simulink model "BLDCMODELTOTALNEURON"  (R2020a)
settings: Solver=ode45  StartTime=0.0  StopTime=2  RelTol=1e-3  EnableMultiTasking=on
InitFcn:
  | clc;
StopFcn:
  | clc;
undefined symbols (not defined in the file): sigbuilder_block, Ts
libraries: neural x55, fl_lib x14, nesl_utility x14, simulink x7, spsIGBTDiodeLib x6, spsVoltageMeasurementLib x3, powerlib_extras x1, spsControlledVoltageSourceLib x1, spsGroundLib x1, spsThreePhaseVIMeasurementLib x1, spspowerguiLib x1
(part 2 of 3)

== system BLDCMODELTOTALNEURON/BLDC Model/emf generation/Phase c ==
  note: Phi' r
  the,we : Inport
  Demux : Demux  Outputs=2
      settings: DisplayOption=none
  Gain4 : Gain  Gain=0.175  SaturateOnIntegerOverflow=on  OutDataTypeStr=Inherit: Same as input  ParamDataTypeStr=Inherit: Same as input
  Product1 : Product  SaturateOnIntegerOverflow=on  OutDataTypeStr=Inherit: Same as first input
  cos (u(1)) : Subsystem
  phi'r : Outport
  E : Outport  Port=2
  wires:
  Gain4/1 -> Product1/1, phi'r/1
  Product1/1 -> E/1
  the,we/1 -> Demux/1
  Demux/2 -> Product1/2
  Demux/1 -> cos (u(1))/1(In1)
  cos (u(1))/1(Out1) -> Gain4/1

== system BLDCMODELTOTALNEURON/Function Fitting Neural Network/Layer 1/Delays 1 ==
  "p{1}" : Inport  PortDimensions=9
      mask Display: e = 0.06;c1 = [120 230 180]/255;c2 = ([120 230 180]+0)/(256+128);c3 = ([120 230 180]+128)/(256+128);patch([0 1 1 0],[0 0 1 1],c1);patch([0 1 1 1-e 1-e 0+e],[0 0 1 1-e 0+e 0+e],c2);patch([0 0 1 1-e 0+e 0+e],[0 1 1 1-e 1-e 0+e],c3);plot([0 1 1 0 0],[0 0 1 1 0]);
  mux : Mux  Inputs=1
      mask Display: e = 0.06;c1 = [120 150 230]/255;c2 = ([120 150 230]+0)/383;c3 = ([120 150 230]+128)/383;patch([0 1 1 0],[0 0 1 1],c1);patch([0 1 1 1-e 1-e 0+e],[0 0 1 1-e 0+e 0+e],c2);patch([0 0 1 1-e 0+e 0+e],[0 1 1 1-e 1-e 0+e],c3);plot([0 1 1 0 0],[0 0 1 1 0]);disp('Mux')
  "pd{1,1}" : Outport
      mask Display: e = 0.06;c1 = [120 230 180]/255;c2 = ([120 230 180]+0)/(256+128);c3 = ([120 230 180]+128)/(256+128);patch([0 1 1 0],[0 0 1 1],c1);patch([0 1 1 1-e 1-e 0+e],[0 0 1 1-e 0+e 0+e],c2);patch([0 0 1 1-e 0+e 0+e],[0 1 1 1-e 1-e 0+e],c3);plot([0 1 1 0 0],[0 0 1 1 0]);
  wires:
  "p{1}"/1 -> mux/1
  mux/1 -> "pd{1,1}"/1

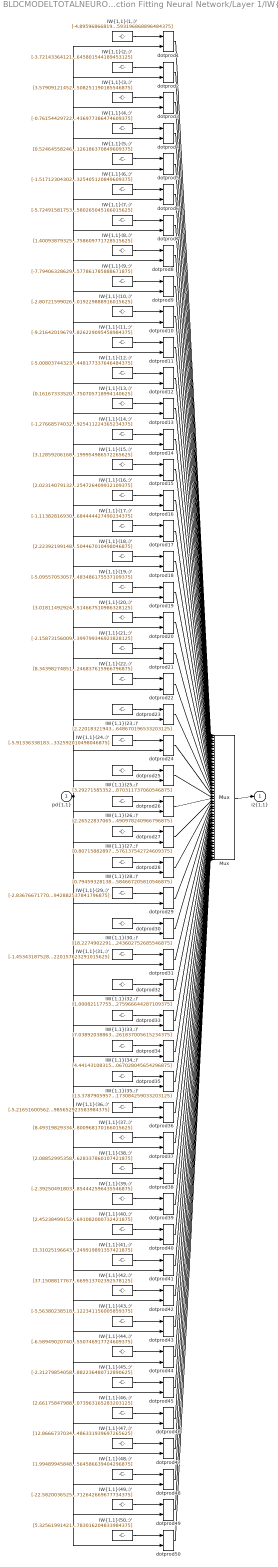
== system BLDCMODELTOTALNEURON/Function Fitting Neural Network/Layer 1/IW{1,1} ==
  "pd{1,1}" : Inport  PortDimensions=9
      mask Display: e = 0.06;c1 = [120 230 180]/255;c2 = ([120 230 180]+0)/(256+128);c3 = ([120 230 180]+128)/(256+128);patch([0 1 1 0],[0 0 1 1],c1);patch([0 1 1 1-e 1-e 0+e],[0 0 1 1-e 0+e 0+e],c2);patch([0 0 1 1-e 0+e 0+e],[0 1 1 1-e 1-e 0+e],c3);plot([0 1 1 0 0],[0 0 1 1 0]);
  "IW{1,1}(1,:)'" : Constant  Value=[-4.895968668193777517672060639597475528717041015625;5.40347313688422303812330937944352626800537109375;2.74044730962565186160873054177500307559967041015625;2.61285690437117157358670738176442682743072509765625;-8.18219538608644114674461889080703258514404296875;5.37405300526213380862827762030065059661865234375;-2.547081241809125540243030627607367932796478271484375;-7.45222912554785299477089210995472967624664306640625;2.3353386247630023575538871227763593196868896484375]
      mask Display: e = 0.06;c1 = [120 150 230]/255;c2 = ([120 150 230]+0)/383;c3 = ([120 150 230]+128)/383;patch([0 1 1 0],[0 0 1 1],c1);patch([0 1 1 1-e 1-e 0+e],[0 0 1 1-e 0+e 0+e],c2);patch([0 0 1 1-e 0+e 0+e],[0 1 1 1-e 1-e 0+e],c3);plot([0 1 1 0 0],[0 0 1 1 0]);disp('Weights');
  "IW{1,1}(10,:)'" : Constant  Value=[-2.807215990265720773066959736752323806285858154296875;0.53318125450332398695962865531328134238719940185546875;1.73233750776441564056540300953201949596405029296875;-6.7636512082147479674176793196238577365875244140625;6.88789031656800165848153483239002525806427001953125;-1.1843020529516923300406006092089228332042694091796875;1.77424013763668231291603660793043673038482666015625;7.99713610623197279636542589287273585796356201171875;0.447326594167716307115512108794064261019229888916015625]
      mask Display: e = 0.06;c1 = [120 150 230]/255;c2 = ([120 150 230]+0)/383;c3 = ([120 150 230]+128)/383;patch([0 1 1 0],[0 0 1 1],c1);patch([0 1 1 1-e 1-e 0+e],[0 0 1 1-e 0+e 0+e],c2);patch([0 0 1 1-e 0+e 0+e],[0 1 1 1-e 1-e 0+e],c3);plot([0 1 1 0 0],[0 0 1 1 0]);disp('Weights');
  "IW{1,1}(11,:)'" : Constant  Value=[-9.216420196795439778725267387926578521728515625;7.1594195626589272052342494134791195392608642578125;3.118246074238363529929074502433650195598602294921875;0.74384522324622814881678323217784054577350616455078125;-2.420490963926231753333695451146923005580902099609375;5.44455711163404476593541403417475521564483642578125;3.547825214125399639897295855917036533355712890625;4.30621318872842895331132240244187414646148681640625;1.096405026223636891558044226258061826229095458984375]
      mask Display: e = 0.06;c1 = [120 150 230]/255;c2 = ([120 150 230]+0)/383;c3 = ([120 150 230]+128)/383;patch([0 1 1 0],[0 0 1 1],c1);patch([0 1 1 1-e 1-e 0+e],[0 0 1 1-e 0+e 0+e],c2);patch([0 0 1 1-e 0+e 0+e],[0 1 1 1-e 1-e 0+e],c3);plot([0 1 1 0 0],[0 0 1 1 0]);disp('Weights');
  "IW{1,1}(12,:)'" : Constant  Value=[-5.00803744323493038592687298660166561603546142578125;5.9761920590233188477213843725621700286865234375;0.320001378281075166132296772047993727028369903564453125;-2.738915566294051640028328620246611535549163818359375;1.0574131975688112472511193118407391011714935302734375;11.1576349013176656654877660912461578845977783203125;10.25816732987643575825131847523152828216552734375;5.71739885726999741422105216770432889461517333984375;0.52981483115273331208072704612277448177337646484375]
      mask Display: e = 0.06;c1 = [120 150 230]/255;c2 = ([120 150 230]+0)/383;c3 = ([120 150 230]+128)/383;patch([0 1 1 0],[0 0 1 1],c1);patch([0 1 1 1-e 1-e 0+e],[0 0 1 1-e 0+e 0+e],c2);patch([0 0 1 1-e 0+e 0+e],[0 1 1 1-e 1-e 0+e],c3);plot([0 1 1 0 0],[0 0 1 1 0]);disp('Weights');
  "IW{1,1}(13,:)'" : Constant  Value=[0.1616733352080349794821501063779578544199466705322265625;-1.90626528235715131387451037880964577198028564453125;1.1517495220095372854274273777264170348644256591796875;-1.468598245944300106913260606233961880207061767578125;-6.27844796813521188738604905665852129459381103515625;3.5109383197600099180135657661594450473785400390625;-3.687189907329767368793227433343417942523956298828125;-1.6200010345593092164762083484674803912639617919921875;2.260455325759112898964531268575228750705718994140625]
      mask Display: e = 0.06;c1 = [120 150 230]/255;c2 = ([120 150 230]+0)/383;c3 = ([120 150 230]+128)/383;patch([0 1 1 0],[0 0 1 1],c1);patch([0 1 1 1-e 1-e 0+e],[0 0 1 1-e 0+e 0+e],c2);patch([0 0 1 1-e 0+e 0+e],[0 1 1 1-e 1-e 0+e],c3);plot([0 1 1 0 0],[0 0 1 1 0]);disp('Weights');
  "IW{1,1}(14,:)'" : Constant  Value=[-1.2766857403284517236130568562657572329044342041015625;-5.73369882955798715329365222714841365814208984375;3.227374843555661954042079742066562175750732421875;-7.7809955575162117469290024018846452236175537109375;2.80775474671538471937992653693072497844696044921875;-4.3767986431355172527446484309621155261993408203125;7.8290605045435910369633347727358341217041015625;6.4679041165319812733969229157082736492156982421875;-3.894484835375331410745047833188436925411224365234375]
      mask Display: e = 0.06;c1 = [120 150 230]/255;c2 = ([120 150 230]+0)/383;c3 = ([120 150 230]+128)/383;patch([0 1 1 0],[0 0 1 1],c1);patch([0 1 1 1-e 1-e 0+e],[0 0 1 1-e 0+e 0+e],c2);patch([0 0 1 1-e 0+e 0+e],[0 1 1 1-e 1-e 0+e],c3);plot([0 1 1 0 0],[0 0 1 1 0]);disp('Weights');
  "IW{1,1}(15,:)'" : Constant  Value=[3.1285920616828253315588881378062069416046142578125;2.81705887052771064560374725260771811008453369140625;-3.887956696466934314315722076571546494960784912109375;5.02906629611409972113733601872809231281280517578125;0.6170228014013081629940415950841270387172698974609375;4.6865213003801642344114952720701694488525390625;-8.101108360563227250850104610435664653778076171875;-4.9140036575473029500926713808439671993255615234375;4.058733138775412641052753315307199954986572265625]
      mask Display: e = 0.06;c1 = [120 150 230]/255;c2 = ([120 150 230]+0)/383;c3 = ([120 150 230]+128)/383;patch([0 1 1 0],[0 0 1 1],c1);patch([0 1 1 1-e 1-e 0+e],[0 0 1 1-e 0+e 0+e],c2);patch([0 0 1 1-e 0+e 0+e],[0 1 1 1-e 1-e 0+e],c3);plot([0 1 1 0 0],[0 0 1 1 0]);disp('Weights');
  "IW{1,1}(16,:)'" : Constant  Value=[2.023140791325761522756465637939982116222381591796875;3.199313205814582783403920984710566699504852294921875;-3.629430220216549596301547353505156934261322021484375;2.30078335496623598288579159998334944248199462890625;-3.870890427542229783597349523915909230709075927734375;2.513060115012128559186521670198999345302581787109375;-2.583375254625132289021394171868450939655303955078125;-4.177607392620398485405530664138495922088623046875;-0.476403165367220216008803390650427900254726409912109375]
      mask Display: e = 0.06;c1 = [120 150 230]/255;c2 = ([120 150 230]+0)/383;c3 = ([120 150 230]+128)/383;patch([0 1 1 0],[0 0 1 1],c1);patch([0 1 1 1-e 1-e 0+e],[0 0 1 1-e 0+e 0+e],c2);patch([0 0 1 1-e 0+e 0+e],[0 1 1 1-e 1-e 0+e],c3);plot([0 1 1 0 0],[0 0 1 1 0]);disp('Weights');
  "IW{1,1}(17,:)'" : Constant  Value=[-1.113828169301168458105166791938245296478271484375;1.1778404473012773490125937314587645232677459716796875;1.620901404126910971825736851315014064311981201171875;-1.766146228500121484472629163064993917942047119140625;0.646115936343579999601161034661345183849334716796875;1.66630542385350910450370065518654882907867431640625;1.2524116425207412195419465206214226782321929931640625;0.8812841366291574995983637563767842948436737060546875;2.343840383667620042018597814603708684444427490234375]
      mask Display: e = 0.06;c1 = [120 150 230]/255;c2 = ([120 150 230]+0)/383;c3 = ([120 150 230]+128)/383;patch([0 1 1 0],[0 0 1 1],c1);patch([0 1 1 1-e 1-e 0+e],[0 0 1 1-e 0+e 0+e],c2);patch([0 0 1 1-e 0+e 0+e],[0 1 1 1-e 1-e 0+e],c3);plot([0 1 1 0 0],[0 0 1 1 0]);disp('Weights');
  "IW{1,1}(18,:)'" : Constant  Value=[2.223921991486593530140680741169489920139312744140625;-0.054825426871896072722467607718499493785202503204345703125;0.0022185476097710652050587487593702462618239223957061767578125;-0.5843966860481921710146480108960531651973724365234375;3.799990339256197557915584184229373931884765625;-1.9218355438914278554562997669563628733158111572265625;-3.537447672391386799262136264587752521038055419921875;-1.0586896092735147423269381761201657354831695556640625;2.684374086787240099027940232190303504467010498046875]
      mask Display: e = 0.06;c1 = [120 150 230]/255;c2 = ([120 150 230]+0)/383;c3 = ([120 150 230]+128)/383;patch([0 1 1 0],[0 0 1 1],c1);patch([0 1 1 1-e 1-e 0+e],[0 0 1 1-e 0+e 0+e],c2);patch([0 0 1 1-e 0+e 0+e],[0 1 1 1-e 1-e 0+e],c3);plot([0 1 1 0 0],[0 0 1 1 0]);disp('Weights');
  "IW{1,1}(19,:)'" : Constant  Value=[-5.0955705305759071421789485611952841281890869140625;6.05178194090348053890693336143158376216888427734375;-1.491669072534929085804833448491990566253662109375;-0.94100410130936185115757552921422757208347320556640625;-1.6970243036780334744406673053163103759288787841796875;-2.266366636401446754689459339715540409088134765625;-3.1732804450517395622455296688713133335113525390625;2.774317765718105288641481820377521216869354248046875;1.1986759118675640589657405143952928483486175537109375]
      mask Display: e = 0.06;c1 = [120 150 230]/255;c2 = ([120 150 230]+0)/383;c3 = ([120 150 230]+128)/383;patch([0 1 1 0],[0 0 1 1],c1);patch([0 1 1 1-e 1-e 0+e],[0 0 1 1-e 0+e 0+e],c2);patch([0 0 1 1-e 0+e 0+e],[0 1 1 1-e 1-e 0+e],c3);plot([0 1 1 0 0],[0 0 1 1 0]);disp('Weights');
  "IW{1,1}(2,:)'" : Constant  Value=[-3.7214336412183417479582203668542206287384033203125;8.4268142416087190582629773416556417942047119140625;-3.02879148438673073684412884176708757877349853515625;0.2284576077078076250526095236637047491967678070068359375;1.005184022489817419199198411661200225353240966796875;4.73916034710702316345987128443084657192230224609375;2.513388967630310499856705064303241670131683349609375;-2.5965278619095233381131038186140358448028564453125;-4.3974879944557887512246452388353645801544189453125]
      mask Display: e = 0.06;c1 = [120 150 230]/255;c2 = ([120 150 230]+0)/383;c3 = ([120 150 230]+128)/383;patch([0 1 1 0],[0 0 1 1],c1);patch([0 1 1 1-e 1-e 0+e],[0 0 1 1-e 0+e 0+e],c2);patch([0 0 1 1-e 0+e 0+e],[0 1 1 1-e 1-e 0+e],c3);plot([0 1 1 0 0],[0 0 1 1 0]);disp('Weights');
  "IW{1,1}(20,:)'" : Constant  Value=[3.01811492924852498020982238813303411006927490234375;-3.62725956127743831558518650126643478870391845703125;-1.842623857170338386168850774993188679218292236328125;-5.19975075112496920581861559185199439525604248046875;1.966417547133222143429520656354725360870361328125;0.2434354388569480998061322907233261503279209136962890625;8.19305073136916917064809240400791168212890625;0.87614260508461594412210615701042115688323974609375;-0.89756050648464213992383520235307514667510986328125]
      mask Display: e = 0.06;c1 = [120 150 230]/255;c2 = ([120 150 230]+0)/383;c3 = ([120 150 230]+128)/383;patch([0 1 1 0],[0 0 1 1],c1);patch([0 1 1 1-e 1-e 0+e],[0 0 1 1-e 0+e 0+e],c2);patch([0 0 1 1-e 0+e 0+e],[0 1 1 1-e 1-e 0+e],c3);plot([0 1 1 0 0],[0 0 1 1 0]);disp('Weights');
  "IW{1,1}(21,:)'" : Constant  Value=[-2.158731560096526447267706316779367625713348388671875;-0.8746332604844859748283170119975693523883819580078125;3.05676503556049272702921371092088520526885986328125;3.081958001652896239619394691544584929943084716796875;-6.09089804270805057484494682285003364086151123046875;-1.5170091317769973660034565909882076084613800048828125;2.515311414585273297461753827519714832305908203125;-1.51894932821134087674863621941767632961273193359375;4.67491695196711010140688813407905399799346923828125]
      mask Display: e = 0.06;c1 = [120 150 230]/255;c2 = ([120 150 230]+0)/383;c3 = ([120 150 230]+128)/383;patch([0 1 1 0],[0 0 1 1],c1);patch([0 1 1 1-e 1-e 0+e],[0 0 1 1-e 0+e 0+e],c2);patch([0 0 1 1-e 0+e 0+e],[0 1 1 1-e 1-e 0+e],c3);plot([0 1 1 0 0],[0 0 1 1 0]);disp('Weights');
  "IW{1,1}(22,:)'" : Constant  Value=[8.343982748517642988872466958127915859222412109375;-2.161196645266016513886597749660722911357879638671875;-3.9544004180846030749307828955352306365966796875;-2.43457845164129249582174452370963990688323974609375;-5.205305155843110043178967316634953022003173828125;1.0130992099416860074967416949220933020114898681640625;6.34578855801143770776207020389847457408905029296875;2.20944537619115966009530893643386662006378173828125;-0.484853150291399248583701364623266272246837615966796875]
      mask Display: e = 0.06;c1 = [120 150 230]/255;c2 = ([120 150 230]+0)/383;c3 = ([120 150 230]+128)/383;patch([0 1 1 0],[0 0 1 1],c1);patch([0 1 1 1-e 1-e 0+e],[0 0 1 1-e 0+e 0+e],c2);patch([0 0 1 1-e 0+e 0+e],[0 1 1 1-e 1-e 0+e],c3);plot([0 1 1 0 0],[0 0 1 1 0]);disp('Weights');
  "IW{1,1}(23,:)'" : Constant  Value=[2.22018321943891461245357277221046388149261474609375;-1.8800292969605318926795689549180679023265838623046875;-2.243768721796227882947505349875427782535552978515625;-1.057276982754526084562485266360454261302947998046875;-1.2433812829791133225398880313150584697723388671875;-1.383969860461479850499699750798754394054412841796875;3.058730398982790976702972329803742468357086181640625;0.53913955545679181913243382950895465910434722900390625;0.1595438162536411408343184348268550820648670196533203125]
      mask Display: e = 0.06;c1 = [120 150 230]/255;c2 = ([120 150 230]+0)/383;c3 = ([120 150 230]+128)/383;patch([0 1 1 0],[0 0 1 1],c1);patch([0 1 1 1-e 1-e 0+e],[0 0 1 1-e 0+e 0+e],c2);patch([0 0 1 1-e 0+e 0+e],[0 1 1 1-e 1-e 0+e],c3);plot([0 1 1 0 0],[0 0 1 1 0]);disp('Weights');
  "IW{1,1}(24,:)'" : Constant  Value=[-5.9133633818331219345054705627262592315673828125;7.325130508331572087854510755278170108795166015625;0.67854478523987860061339461026364006102085113525390625;-5.54971457443748494853252850589342415332794189453125;2.338297073162864503359514856128953397274017333984375;-4.82297855274858289220674123498611152172088623046875;4.53075163897600052820280325249768793582916259765625;7.4605392659156422041633049957454204559326171875;-0.129756839337727025718294271428021602332592010498046875]
      mask Display: e = 0.06;c1 = [120 150 230]/255;c2 = ([120 150 230]+0)/383;c3 = ([120 150 230]+128)/383;patch([0 1 1 0],[0 0 1 1],c1);patch([0 1 1 1-e 1-e 0+e],[0 0 1 1-e 0+e 0+e],c2);patch([0 0 1 1-e 0+e 0+e],[0 1 1 1-e 1-e 0+e],c3);plot([0 1 1 0 0],[0 0 1 1 0]);disp('Weights');
  "IW{1,1}(25,:)'" : Constant  Value=[3.2927158535273175488100605434738099575042724609375;-7.466663455404482618860129150561988353729248046875;1.859971234331494915892335484386421740055084228515625;-4.40535563617537917480149189941585063934326171875;-1.4389465848187310559325169379008002579212188720703125;-7.14086549853874519300234169350005686283111572265625;13.11373443627413593048913753591477870941162109375;2.926398481880311042147013722569681704044342041015625;-4.11809256079247898441053621354512870311737060546875]
      mask Display: e = 0.06;c1 = [120 150 230]/255;c2 = ([120 150 230]+0)/383;c3 = ([120 150 230]+128)/383;patch([0 1 1 0],[0 0 1 1],c1);patch([0 1 1 1-e 1-e 0+e],[0 0 1 1-e 0+e 0+e],c2);patch([0 0 1 1-e 0+e 0+e],[0 1 1 1-e 1-e 0+e],c3);plot([0 1 1 0 0],[0 0 1 1 0]);disp('Weights');
  "IW{1,1}(26,:)'" : Constant  Value=[2.26522837065874060868964079418219625949859619140625;4.2525822507105086600631693727336823940277099609375;-4.61264142259110609955996551434509456157684326171875;-6.31738226144889036817176020122133195400238037109375;5.23253833887288255510839007911272346973419189453125;-8.962684825422229550895281136035919189453125;-5.88140626410156119874272917513735592365264892578125;6.1683261761612886431294100475497543811798095703125;-5.83295418242180829793142038397490978240966796875]
      mask Display: e = 0.06;c1 = [120 150 230]/255;c2 = ([120 150 230]+0)/383;c3 = ([120 150 230]+128)/383;patch([0 1 1 0],[0 0 1 1],c1);patch([0 1 1 1-e 1-e 0+e],[0 0 1 1-e 0+e 0+e],c2);patch([0 0 1 1-e 0+e 0+e],[0 1 1 1-e 1-e 0+e],c3);plot([0 1 1 0 0],[0 0 1 1 0]);disp('Weights');
  "IW{1,1}(27,:)'" : Constant  Value=[0.80715882897217128277844722106237895786762237548828125;-1.5342936386238827939365592101239599287509918212890625;-0.42012466949483495692874157612095586955547332763671875;-8.11645473537303274724763468839228153228759765625;-1.1314757465724880614033054371247999370098114013671875;14.781667595466473130727536045014858245849609375;1.8109771676627250958091508437064476311206817626953125;3.9085959869213322548375799669884145259857177734375;-6.07921746579665178700224714702926576137542724609375]
      mask Display: e = 0.06;c1 = [120 150 230]/255;c2 = ([120 150 230]+0)/383;c3 = ([120 150 230]+128)/383;patch([0 1 1 0],[0 0 1 1],c1);patch([0 1 1 1-e 1-e 0+e],[0 0 1 1-e 0+e 0+e],c2);patch([0 0 1 1-e 0+e 0+e],[0 1 1 1-e 1-e 0+e],c3);plot([0 1 1 0 0],[0 0 1 1 0]);disp('Weights');
  "IW{1,1}(28,:)'" : Constant  Value=[0.79459328138242157901771633987664245069026947021484375;-1.8079929837847250606586158028221689164638519287109375;1.69049420812355766230439257924444973468780517578125;-0.73313934220313348166797595695243217051029205322265625;-1.5224778868556130273503868011175654828548431396484375;0.4887267103351027319746435750857926905155181884765625;3.311316422988955121553544813650660216808319091796875;0.575415043139363202584490863955579698085784912109375;-3.7366302997256735096698321285657584667205810546875]
      mask Display: e = 0.06;c1 = [120 150 230]/255;c2 = ([120 150 230]+0)/383;c3 = ([120 150 230]+128)/383;patch([0 1 1 0],[0 0 1 1],c1);patch([0 1 1 1-e 1-e 0+e],[0 0 1 1-e 0+e 0+e],c2);patch([0 0 1 1-e 0+e 0+e],[0 1 1 1-e 1-e 0+e],c3);plot([0 1 1 0 0],[0 0 1 1 0]);disp('Weights');
  "IW{1,1}(29,:)'" : Constant  Value=[-2.83676671770210919731880494509823620319366455078125;3.78002105566060198071909326245076954364776611328125;-2.323486567515789857907293480820953845977783203125;-0.95512967653330071993167393884505145251750946044921875;-0.60568244848216823417175191934802569448947906494140625;2.210703505491417697470524217351339757442474365234375;-2.039411367259091445447438672999851405620574951171875;-0.73412589888445289876273136542295105755329132080078125;-1.7846661191017278991211014727014116942882537841796875]
      mask Display: e = 0.06;c1 = [120 150 230]/255;c2 = ([120 150 230]+0)/383;c3 = ([120 150 230]+128)/383;patch([0 1 1 0],[0 0 1 1],c1);patch([0 1 1 1-e 1-e 0+e],[0 0 1 1-e 0+e 0+e],c2);patch([0 0 1 1-e 0+e 0+e],[0 1 1 1-e 1-e 0+e],c3);plot([0 1 1 0 0],[0 0 1 1 0]);disp('Weights');
  "IW{1,1}(3,:)'" : Constant  Value=[3.579091214525738084972772412584163248538970947265625;-2.431777730337249199266125287977047264575958251953125;-1.4837016201098738310548696972546167671680450439453125;3.025023954173181817139948179828934371471405029296875;-5.09547170650127778657179078436456620693206787109375;-4.7348999293881117722548879100941121578216552734375;-0.428598247009314980981997678100015036761760711669921875;-3.530088208951525086121137064765207469463348388671875;8.6702058743657044459496319177560508251190185546875]
      mask Display: e = 0.06;c1 = [120 150 230]/255;c2 = ([120 150 230]+0)/383;c3 = ([120 150 230]+128)/383;patch([0 1 1 0],[0 0 1 1],c1);patch([0 1 1 1-e 1-e 0+e],[0 0 1 1-e 0+e 0+e],c2);patch([0 0 1 1-e 0+e 0+e],[0 1 1 1-e 1-e 0+e],c3);plot([0 1 1 0 0],[0 0 1 1 0]);disp('Weights');
  "IW{1,1}(30,:)'" : Constant  Value=[18.2274902291847951119052595458924770355224609375;0.10029042444976567216574636631776229478418827056884765625;-15.2216980933245960017075049108825623989105224609375;-51.1700178399161842435205471701920032501220703125;-56.02455973781388109955514664761722087860107421875;47.243740956707284794902079738676548004150390625;10.6716383101642922071050634258426725864410400390625;27.839487972618687905423939810134470462799072265625;-6.3769331352299314374931782367639243602752685546875]
      mask Display: e = 0.06;c1 = [120 150 230]/255;c2 = ([120 150 230]+0)/383;c3 = ([120 150 230]+128)/383;patch([0 1 1 0],[0 0 1 1],c1);patch([0 1 1 1-e 1-e 0+e],[0 0 1 1-e 0+e 0+e],c2);patch([0 0 1 1-e 0+e 0+e],[0 1 1 1-e 1-e 0+e],c3);plot([0 1 1 0 0],[0 0 1 1 0]);disp('Weights');
  "IW{1,1}(31,:)'" : Constant  Value=[-1.4534318752841068889125608620815910398960113525390625;6.1247562160562427635568383266218006610870361328125;-2.8918337539965239813000152935273945331573486328125;0.9028102978327281480375177125097252428531646728515625;-4.3042053734154190891558755538426339626312255859375;-1.845935973018257403310826703091152012348175048828125;2.573811245121011115344344943878240883350372314453125;-3.919961580962290526031210902146995067596435546875;2.665708563941960651533236159593798220157623291015625]
      mask Display: e = 0.06;c1 = [120 150 230]/255;c2 = ([120 150 230]+0)/383;c3 = ([120 150 230]+128)/383;patch([0 1 1 0],[0 0 1 1],c1);patch([0 1 1 1-e 1-e 0+e],[0 0 1 1-e 0+e 0+e],c2);patch([0 0 1 1-e 0+e 0+e],[0 1 1 1-e 1-e 0+e],c3);plot([0 1 1 0 0],[0 0 1 1 0]);disp('Weights');
  "IW{1,1}(32,:)'" : Constant  Value=[1.000821177556808994069115215097554028034210205078125;-1.1601853380740809740245822467841207981109619140625;-1.2470947311945967950208569163805805146694183349609375;-1.288548983066672537489694150281138718128204345703125;1.099069146087539028400215102010406553745269775390625;-2.518438507999196218634097022004425525665283203125;7.2023214000541369017582837841473519802093505859375;5.20235982672458963094186401576735079288482666015625;-1.8693746816614795758226819089031778275966644287109375]
      mask Display: e = 0.06;c1 = [120 150 230]/255;c2 = ([120 150 230]+0)/383;c3 = ([120 150 230]+128)/383;patch([0 1 1 0],[0 0 1 1],c1);patch([0 1 1 1-e 1-e 0+e],[0 0 1 1-e 0+e 0+e],c2);patch([0 0 1 1-e 0+e 0+e],[0 1 1 1-e 1-e 0+e],c3);plot([0 1 1 0 0],[0 0 1 1 0]);disp('Weights');
  "IW{1,1}(33,:)'" : Constant  Value=[7.03892038863087776690008467994630336761474609375;-11.064903976837282328915534890256822109222412109375;0.69971359527199628036697731658932752907276153564453125;-6.25767087593949344892507724580354988574981689453125;1.2295683633822871438923129971954040229320526123046875;-22.917965838783505461151435156352818012237548828125;-0.1913542269049568200767197367895278148353099822998046875;-17.30670372769272802315754233859479427337646484375;-9.9208972492461295900056938990019261837005615234375]
      mask Display: e = 0.06;c1 = [120 150 230]/255;c2 = ([120 150 230]+0)/383;c3 = ([120 150 230]+128)/383;patch([0 1 1 0],[0 0 1 1],c1);patch([0 1 1 1-e 1-e 0+e],[0 0 1 1-e 0+e 0+e],c2);patch([0 0 1 1-e 0+e 0+e],[0 1 1 1-e 1-e 0+e],c3);plot([0 1 1 0 0],[0 0 1 1 0]);disp('Weights');
  "IW{1,1}(34,:)'" : Constant  Value=[4.44143108315375911843148060142993927001953125;1.5265309562414410837760669892304576933383941650390625;-4.78652973989852625891217030584812164306640625;2.7260670293901849703388506895862519741058349609375;-0.1258984760152474235983532935279072262346744537353515625;1.6425137964559730630043077326263301074504852294921875;-0.026399067741740452064380662022813339717686176300048828125;-0.268992813793498763974554321976029314100742340087890625;4.02828486418141817893001643824391067028045654296875]
      mask Display: e = 0.06;c1 = [120 150 230]/255;c2 = ([120 150 230]+0)/383;c3 = ([120 150 230]+128)/383;patch([0 1 1 0],[0 0 1 1],c1);patch([0 1 1 1-e 1-e 0+e],[0 0 1 1-e 0+e 0+e],c2);patch([0 0 1 1-e 0+e 0+e],[0 1 1 1-e 1-e 0+e],c3);plot([0 1 1 0 0],[0 0 1 1 0]);disp('Weights');
  "IW{1,1}(35,:)'" : Constant  Value=[13.378790595756438364105633809231221675872802734375;-1.5596846444388201557984530154499225318431854248046875;-8.8549881877569429633467734674923121929168701171875;0.278641989673728718290846018135198391973972320556640625;-2.218723650480382669769596759579144418239593505859375;2.3815327462113042855662570218555629253387451171875;4.3910483195623868368784314952790737152099609375;-1.856289349292984613981616348610259592533111572265625;1.2448266838758588193059040349908173084259033203125]
      mask Display: e = 0.06;c1 = [120 150 230]/255;c2 = ([120 150 230]+0)/383;c3 = ([120 150 230]+128)/383;patch([0 1 1 0],[0 0 1 1],c1);patch([0 1 1 1-e 1-e 0+e],[0 0 1 1-e 0+e 0+e],c2);patch([0 0 1 1-e 0+e 0+e],[0 1 1 1-e 1-e 0+e],c3);plot([0 1 1 0 0],[0 0 1 1 0]);disp('Weights');
  "IW{1,1}(36,:)'" : Constant  Value=[-5.2165160056228447871262687840498983860015869140625;3.4932935304848200530614121817052364349365234375;1.349201861956220938054684665985405445098876953125;2.677603341351294741201627402915619313716888427734375;-5.7714083461349314774224694701842963695526123046875;11.9309452097577963769481357303448021411895751953125;1.6614186756337654404802606222801841795444488525390625;-2.04637997400443083506615948863327503204345703125;9.876390703280971905542173772118985652923583984375]
      mask Display: e = 0.06;c1 = [120 150 230]/255;c2 = ([120 150 230]+0)/383;c3 = ([120 150 230]+128)/383;patch([0 1 1 0],[0 0 1 1],c1);patch([0 1 1 1-e 1-e 0+e],[0 0 1 1-e 0+e 0+e],c2);patch([0 0 1 1-e 0+e 0+e],[0 1 1 1-e 1-e 0+e],c3);plot([0 1 1 0 0],[0 0 1 1 0]);disp('Weights');
  "IW{1,1}(37,:)'" : Constant  Value=[8.4931982933498186838505716877989470958709716796875;-2.991790861709237692167562272516079246997833251953125;-6.7006468660041331730781166697852313518524169921875;5.66684323427097513814487683703191578388214111328125;-7.57120136002534582786438477342016994953155517578125;-2.29115809411889781443960600881837308406829833984375;-9.716557655800205139939862419851124286651611328125;-6.75121978701695812929983731009997427463531494140625;4.07104828485823677652888363809324800968170166015625]
      mask Display: e = 0.06;c1 = [120 150 230]/255;c2 = ([120 150 230]+0)/383;c3 = ([120 150 230]+128)/383;patch([0 1 1 0],[0 0 1 1],c1);patch([0 1 1 1-e 1-e 0+e],[0 0 1 1-e 0+e 0+e],c2);patch([0 0 1 1-e 0+e 0+e],[0 1 1 1-e 1-e 0+e],c3);plot([0 1 1 0 0],[0 0 1 1 0]);disp('Weights');
  "IW{1,1}(38,:)'" : Constant  Value=[2.088529953586264920062376404530368745326995849609375;-2.450704266549707188715956363012082874774932861328125;-2.33829321932056632959984199260361492633819580078125;6.7288336579490195532571306102909147739410400390625;-5.49061267695196786320366300060413777828216552734375;1.2500294480874185598651138207060284912586212158203125;0.08831491119464775219061181132929050363600254058837890625;-6.35335261167789067116018486558459699153900146484375;0.2059778279968087211226901445115800015628337860107421875]
      mask Display: e = 0.06;c1 = [120 150 230]/255;c2 = ([120 150 230]+0)/383;c3 = ([120 150 230]+128)/383;patch([0 1 1 0],[0 0 1 1],c1);patch([0 1 1 1-e 1-e 0+e],[0 0 1 1-e 0+e 0+e],c2);patch([0 0 1 1-e 0+e 0+e],[0 1 1 1-e 1-e 0+e],c3);plot([0 1 1 0 0],[0 0 1 1 0]);disp('Weights');
  "IW{1,1}(39,:)'" : Constant  Value=[-2.392504918032547944761745384312234818935394287109375;31.7159889925565181556521565653383731842041015625;-19.035880551040893493563999072648584842681884765625;-2.811650086828039629693876122473739087581634521484375;35.8492056691828793191234581172466278076171875;17.110530804295731144293313263915479183197021484375;23.084408404957553528902280959300696849822998046875;15.093318847338490940046540345065295696258544921875;-3.00479409505088579379616930964402854442596435546875]
      mask Display: e = 0.06;c1 = [120 150 230]/255;c2 = ([120 150 230]+0)/383;c3 = ([120 150 230]+128)/383;patch([0 1 1 0],[0 0 1 1],c1);patch([0 1 1 1-e 1-e 0+e],[0 0 1 1-e 0+e 0+e],c2);patch([0 0 1 1-e 0+e 0+e],[0 1 1 1-e 1-e 0+e],c3);plot([0 1 1 0 0],[0 0 1 1 0]);disp('Weights');
  "IW{1,1}(4,:)'" : Constant  Value=[-0.76154429722584449091726810365798883140087127685546875;-3.865140946642005470579306347644887864589691162109375;2.810067424866792951121396981761790812015533447265625;-2.0679206122518554167299953405745327472686767578125;-0.30951541105722479851891648650052957236766815185546875;3.366032002972835446286126170889474451541900634765625;-0.68917292208956049126555853945319540798664093017578125;-3.91421737785447110269387849257327616214752197265625;-3.855538611321639219653434338397346436977386474609375]
      mask Display: e = 0.06;c1 = [120 150 230]/255;c2 = ([120 150 230]+0)/383;c3 = ([120 150 230]+128)/383;patch([0 1 1 0],[0 0 1 1],c1);patch([0 1 1 1-e 1-e 0+e],[0 0 1 1-e 0+e 0+e],c2);patch([0 0 1 1-e 0+e 0+e],[0 1 1 1-e 1-e 0+e],c3);plot([0 1 1 0 0],[0 0 1 1 0]);disp('Weights');
  "IW{1,1}(40,:)'" : Constant  Value=[2.452384991521587398466408558306284248828887939453125;3.096811057518499499252584428177215158939361572265625;-5.19281998518984710955237460439093410968780517578125;5.6152203407946021940233549685217440128326416015625;-14.72604220900434057739403215236961841583251953125;-4.85256894723468956698297915863804519176483154296875;-3.191000716728321418003133658203296363353729248046875;-4.49492018986455121876133489422500133514404296875;3.58000220958119097502958538825623691082000732421875]
      mask Display: e = 0.06;c1 = [120 150 230]/255;c2 = ([120 150 230]+0)/383;c3 = ([120 150 230]+128)/383;patch([0 1 1 0],[0 0 1 1],c1);patch([0 1 1 1-e 1-e 0+e],[0 0 1 1-e 0+e 0+e],c2);patch([0 0 1 1-e 0+e 0+e],[0 1 1 1-e 1-e 0+e],c3);plot([0 1 1 0 0],[0 0 1 1 0]);disp('Weights');
  "IW{1,1}(41,:)'" : Constant  Value=[3.3102519664394520759742590598762035369873046875;0.473351329623000083302031271159648895263671875;-3.25904259369478932484298638883046805858612060546875;11.7672363405767601562956770067103207111358642578125;6.01052086780126071374752427800558507442474365234375;-12.3251952499961543452400292153470218181610107421875;-1.66113206425894599504999860073439776897430419921875;-6.58785941502866645436142789549194276332855224609375;3.930650713430928089309190909261815249919891357421875]
      mask Display: e = 0.06;c1 = [120 150 230]/255;c2 = ([120 150 230]+0)/383;c3 = ([120 150 230]+128)/383;patch([0 1 1 0],[0 0 1 1],c1);patch([0 1 1 1-e 1-e 0+e],[0 0 1 1-e 0+e 0+e],c2);patch([0 0 1 1-e 0+e 0+e],[0 1 1 1-e 1-e 0+e],c3);plot([0 1 1 0 0],[0 0 1 1 0]);disp('Weights');
  "IW{1,1}(42,:)'" : Constant  Value=[37.150881776758296837215311825275421142578125;-55.18492268530483357835692004300653934478759765625;4.022718820313276211209085886366665363311767578125;-58.673706816738075531247886829078197479248046875;-68.8844313276788255961946561001241207122802734375;58.4727121088444476981749176047742366790771484375;12.7442855762528353125162539072334766387939453125;33.1212786788305635354845435358583927154541015625;-4.8305714832569766059577887062914669513702392578125]
      mask Display: e = 0.06;c1 = [120 150 230]/255;c2 = ([120 150 230]+0)/383;c3 = ([120 150 230]+128)/383;patch([0 1 1 0],[0 0 1 1],c1);patch([0 1 1 1-e 1-e 0+e],[0 0 1 1-e 0+e 0+e],c2);patch([0 0 1 1-e 0+e 0+e],[0 1 1 1-e 1-e 0+e],c3);plot([0 1 1 0 0],[0 0 1 1 0]);disp('Weights');
  "IW{1,1}(43,:)'" : Constant  Value=[-5.56380238518266967417957857833243906497955322265625;0.03352896070247768367522667176672257483005523681640625;3.00512413127854838279517935006879270076751708984375;2.96301586369306857449146264116279780864715576171875;-2.6412629354603467390916193835437297821044921875;7.44659200164256684928432150627486407756805419921875;1.43785634942696560756303369998931884765625;-4.4448581419289663330118855810724198818206787109375;-0.30697986959050849176122710559866391122341156005859375]
      mask Display: e = 0.06;c1 = [120 150 230]/255;c2 = ([120 150 230]+0)/383;c3 = ([120 150 230]+128)/383;patch([0 1 1 0],[0 0 1 1],c1);patch([0 1 1 1-e 1-e 0+e],[0 0 1 1-e 0+e 0+e],c2);patch([0 0 1 1-e 0+e 0+e],[0 1 1 1-e 1-e 0+e],c3);plot([0 1 1 0 0],[0 0 1 1 0]);disp('Weights');
  "IW{1,1}(44,:)'" : Constant  Value=[-6.58949020740030011467069925856776535511016845703125;5.61721173715779809043624482001177966594696044921875;1.413785061834719414264327497221529483795166015625;-2.94818424594639427738229642272926867008209228515625;-6.4549500242106727654345377231948077678680419921875;5.6393397561049045663139622774906456470489501953125;-7.2612943435046712892244613613002002239227294921875;-1.774898637127661604750983315170742571353912353515625;10.668813704219331839340156875550746917724609375]
      mask Display: e = 0.06;c1 = [120 150 230]/255;c2 = ([120 150 230]+0)/383;c3 = ([120 150 230]+128)/383;patch([0 1 1 0],[0 0 1 1],c1);patch([0 1 1 1-e 1-e 0+e],[0 0 1 1-e 0+e 0+e],c2);patch([0 0 1 1-e 0+e 0+e],[0 1 1 1-e 1-e 0+e],c3);plot([0 1 1 0 0],[0 0 1 1 0]);disp('Weights');
  "IW{1,1}(45,:)'" : Constant  Value=[-2.312798540584005468900841151480562984943389892578125;6.3857168294009465370208999956957995891571044921875;-3.05092518908506082908616008353419601917266845703125;-1.340006785269062472565337884589098393917083740234375;-6.1855460161201865076918693375773727893829345703125;4.442638627253320038335004937835037708282470703125;1.1079534415150236181801801649271510541439056396484375;-2.80109440493968175900363348773680627346038818359375;-0.5528487202193625993373871096991933882236480712890625]
      mask Display: e = 0.06;c1 = [120 150 230]/255;c2 = ([120 150 230]+0)/383;c3 = ([120 150 230]+128)/383;patch([0 1 1 0],[0 0 1 1],c1);patch([0 1 1 1-e 1-e 0+e],[0 0 1 1-e 0+e 0+e],c2);patch([0 0 1 1-e 0+e 0+e],[0 1 1 1-e 1-e 0+e],c3);plot([0 1 1 0 0],[0 0 1 1 0]);disp('Weights');
  "IW{1,1}(46,:)'" : Constant  Value=[2.661758479883007399990901831188239157199859619140625;-5.46291685324124731693018475198186933994293212890625;-0.63711373570406693023215893845190294086933135986328125;0.3741446884612227297139952497673220932483673095703125;-2.082093870394800205758656375110149383544921875;0.57463883851576558203788636092212982475757598876953125;-2.998734291191599954373714354005642235279083251953125;0.286672010283718192713564576479257084429264068603515625;1.284669055814316340757841317099519073963165283203125]
      mask Display: e = 0.06;c1 = [120 150 230]/255;c2 = ([120 150 230]+0)/383;c3 = ([120 150 230]+128)/383;patch([0 1 1 0],[0 0 1 1],c1);patch([0 1 1 1-e 1-e 0+e],[0 0 1 1-e 0+e 0+e],c2);patch([0 0 1 1-e 0+e 0+e],[0 1 1 1-e 1-e 0+e],c3);plot([0 1 1 0 0],[0 0 1 1 0]);disp('Weights');
  "IW{1,1}(47,:)'" : Constant  Value=[12.8666737034711591292079901904799044132232666015625;-11.8418045094891635216072245384566485881805419921875;-4.85049176848345720003408132470212876796722412109375;-0.1521501480686227036898117148666642606258392333984375;5.6042873526386589588810238637961447238922119140625;-11.1783085487774389576998146367259323596954345703125;-6.46226256128151188562469542375765740871429443359375;5.52248228334268009831475865212269127368927001953125;-4.96790533595833583291323520825244486331939697265625]
      mask Display: e = 0.06;c1 = [120 150 230]/255;c2 = ([120 150 230]+0)/383;c3 = ([120 150 230]+128)/383;patch([0 1 1 0],[0 0 1 1],c1);patch([0 1 1 1-e 1-e 0+e],[0 0 1 1-e 0+e 0+e],c2);patch([0 0 1 1-e 0+e 0+e],[0 1 1 1-e 1-e 0+e],c3);plot([0 1 1 0 0],[0 0 1 1 0]);disp('Weights');
  "IW{1,1}(48,:)'" : Constant  Value=[1.9948994584804158325397338558104820549488067626953125;0.2181573967888530141134850737216765992343425750732421875;-1.6633958623808016152878508364665322005748748779296875;3.439418352105118259487426257692277431488037109375;-3.813577628945288733319785023923031985759735107421875;8.257900847886364914529622183181345462799072265625;-1.0679742142029955420667874932405538856983184814453125;-5.24209172469266349025929230265319347381591796875;4.812849231438047326037121820263564586639404296875]
      mask Display: e = 0.06;c1 = [120 150 230]/255;c2 = ([120 150 230]+0)/383;c3 = ([120 150 230]+128)/383;patch([0 1 1 0],[0 0 1 1],c1);patch([0 1 1 1-e 1-e 0+e],[0 0 1 1-e 0+e 0+e],c2);patch([0 0 1 1-e 0+e 0+e],[0 1 1 1-e 1-e 0+e],c3);plot([0 1 1 0 0],[0 0 1 1 0]);disp('Weights');
  "IW{1,1}(49,:)'" : Constant  Value=[-22.5820036525644951552749262191355228424072265625;32.84152661184146637651792843826115131378173828125;-2.79452432569914943627509273937903344631195068359375;10.5897130394403671260761257144622504711151123046875;0.9574022316746988447988542247912846505641937255859375;-33.287025005266031030259910039603710174560546875;-7.89751812289360177743446911335922777652740478515625;-14.640554800282689740242858533747494220733642578125;1.8520817330637466824327930225990712642669677734375]
      mask Display: e = 0.06;c1 = [120 150 230]/255;c2 = ([120 150 230]+0)/383;c3 = ([120 150 230]+128)/383;patch([0 1 1 0],[0 0 1 1],c1);patch([0 1 1 1-e 1-e 0+e],[0 0 1 1-e 0+e 0+e],c2);patch([0 0 1 1-e 0+e 0+e],[0 1 1 1-e 1-e 0+e],c3);plot([0 1 1 0 0],[0 0 1 1 0]);disp('Weights');
  "IW{1,1}(5,:)'" : Constant  Value=[0.52464558246217218862028630610438995063304901123046875;1.1840936765667142704927528029656969010829925537109375;-0.5870172690367712053927107263007201254367828369140625;-0.120523263213762665824191344654536806046962738037109375;0.70490827099396791144414464724832214415073394775390625;0.07065238029798716345997178223115042783319950103759765625;-1.399343965903664610550549696199595928192138671875;-0.441537541358235474664439834668883122503757476806640625;0.56014662826499550529746329630143009126186370849609375]
      mask Display: e = 0.06;c1 = [120 150 230]/255;c2 = ([120 150 230]+0)/383;c3 = ([120 150 230]+128)/383;patch([0 1 1 0],[0 0 1 1],c1);patch([0 1 1 1-e 1-e 0+e],[0 0 1 1-e 0+e 0+e],c2);patch([0 0 1 1-e 0+e 0+e],[0 1 1 1-e 1-e 0+e],c3);plot([0 1 1 0 0],[0 0 1 1 0]);disp('Weights');
  "IW{1,1}(50,:)'" : Constant  Value=[5.3256199142182598649242208921350538730621337890625;-11.8530738122641086107478258782066404819488525390625;3.527143955119672380504880493390373885631561279296875;0.77020541798430108837436591784353367984294891357421875;1.790117059455414771917958205449394881725311279296875;6.7769688724986938410665970877744257450103759765625;-0.278656253693321975806185264445957727730274200439453125;1.9219124854153351034113939022063277661800384521484375;-0.97822654016791632525240629547624848783016204833984375]
      mask Display: e = 0.06;c1 = [120 150 230]/255;c2 = ([120 150 230]+0)/383;c3 = ([120 150 230]+128)/383;patch([0 1 1 0],[0 0 1 1],c1);patch([0 1 1 1-e 1-e 0+e],[0 0 1 1-e 0+e 0+e],c2);patch([0 0 1 1-e 0+e 0+e],[0 1 1 1-e 1-e 0+e],c3);plot([0 1 1 0 0],[0 0 1 1 0]);disp('Weights');
  "IW{1,1}(6,:)'" : Constant  Value=[-1.5171230430298139335576479425071738660335540771484375;1.86275900722956233579452600679360330104827880859375;-1.0896520521000869763383889221586287021636962890625;-0.5697864682005608916171013333951123058795928955078125;-7.30279832624464564361232987721450626850128173828125;5.64240237810450206978885034914128482341766357421875;-0.311915207578944642108353946241550147533416748046875;-3.76735501973723163615659359493292868137359619140625;1.8306428815227098194640120709664188325405120849609375]
      mask Display: e = 0.06;c1 = [120 150 230]/255;c2 = ([120 150 230]+0)/383;c3 = ([120 150 230]+128)/383;patch([0 1 1 0],[0 0 1 1],c1);patch([0 1 1 1-e 1-e 0+e],[0 0 1 1-e 0+e 0+e],c2);patch([0 0 1 1-e 0+e 0+e],[0 1 1 1-e 1-e 0+e],c3);plot([0 1 1 0 0],[0 0 1 1 0]);disp('Weights');
  "IW{1,1}(7,:)'" : Constant  Value=[-5.72491581753663769660533944261260330677032470703125;-19.890707229573113323795041651464998722076416015625;16.62991106175423539070834522135555744171142578125;5.59070787842219285579403731389902532100677490234375;-0.0184041350603553095777176196179425460286438465118408203125;-8.080686997869843679609402897767722606658935546875;-2.218592037529357963165921319159679114818572998046875;-5.94501471818164528571060145623050630092620849609375;15.1156598111435673814639812917448580265045166015625]
      mask Display: e = 0.06;c1 = [120 150 230]/255;c2 = ([120 150 230]+0)/383;c3 = ([120 150 230]+128)/383;patch([0 1 1 0],[0 0 1 1],c1);patch([0 1 1 1-e 1-e 0+e],[0 0 1 1-e 0+e 0+e],c2);patch([0 0 1 1-e 0+e 0+e],[0 1 1 1-e 1-e 0+e],c3);plot([0 1 1 0 0],[0 0 1 1 0]);disp('Weights');
  "IW{1,1}(8,:)'" : Constant  Value=[1.4009387932551236044531606239615939557552337646484375;-5.84707714002727385604885057546198368072509765625;2.169317700000679582927887167898006737232208251953125;4.71779674103439194965403657988645136356353759765625;-2.0911184550530510506405335036106407642364501953125;-0.1393208332417232020450370555408881045877933502197265625;-1.398000557227633944279432398616336286067962646484375;-3.2341877031195309655231540091335773468017578125;4.98935784491216427483095685602165758609771728515625]
      mask Display: e = 0.06;c1 = [120 150 230]/255;c2 = ([120 150 230]+0)/383;c3 = ([120 150 230]+128)/383;patch([0 1 1 0],[0 0 1 1],c1);patch([0 1 1 1-e 1-e 0+e],[0 0 1 1-e 0+e 0+e],c2);patch([0 0 1 1-e 0+e 0+e],[0 1 1 1-e 1-e 0+e],c3);plot([0 1 1 0 0],[0 0 1 1 0]);disp('Weights');
  "IW{1,1}(9,:)'" : Constant  Value=[-7.79406328629590117174075203365646302700042724609375;8.9400645208249134299194338382221758365631103515625;0.312889245477898481073708580879610963165760040283203125;3.09333091091537593086968627176247537136077880859375;-7.9134134786868113309310501790605485439300537109375;2.162430323652487995644833063124679028987884521484375;-1.7890812976913268439460580339073203504085540771484375;-2.312342465565176308217587575200013816356658935546875;6.60972439766521091542017529718577861785888671875]
      mask Display: e = 0.06;c1 = [120 150 230]/255;c2 = ([120 150 230]+0)/383;c3 = ([120 150 230]+128)/383;patch([0 1 1 0],[0 0 1 1],c1);patch([0 1 1 1-e 1-e 0+e],[0 0 1 1-e 0+e 0+e],c2);patch([0 0 1 1-e 0+e 0+e],[0 1 1 1-e 1-e 0+e],c3);plot([0 1 1 0 0],[0 0 1 1 0]);disp('Weights');
  Mux : Mux  Inputs=50
      mask Display: e = 0.06;c1 = [120 150 230]/255;c2 = ([120 150 230]+0)/383;c3 = ([120 150 230]+128)/383;patch([0 1 1 0],[0 0 1 1],c1);patch([0 1 1 1-e 1-e 0+e],[0 0 1 1-e 0+e 0+e],c2);patch([0 0 1 1-e 0+e 0+e],[0 1 1 1-e 1-e 0+e],c3);plot([0 1 1 0 0],[0 0 1 1 0]);disp('Mux');
  dotprod{1..50} (50 alike) : neural/Weight Functions/dotprod
  "iz{1,1}" : Outport
      mask Display: e = 0.06;c1 = [120 230 180]/255;c2 = ([120 230 180]+0)/(256+128);c3 = ([120 230 180]+128)/(256+128);patch([0 1 1 0],[0 0 1 1],c1);patch([0 1 1 1-e 1-e 0+e],[0 0 1 1-e 0+e 0+e],c2);patch([0 0 1 1-e 0+e 0+e],[0 1 1 1-e 1-e 0+e],c3);plot([0 1 1 0 0],[0 0 1 1 0]);
  wires:
  "IW{1,1}(1,:)'"/1 -> dotprod1/1
  "pd{1,1}"/1 -> dotprod1/2, dotprod2/2, dotprod3/2, dotprod4/2, dotprod5/2, dotprod6/2, dotprod7/2, dotprod8/2, dotprod9/2, dotprod10/2, dotprod11/2, dotprod12/2, dotprod13/2, dotprod14/2, dotprod15/2, dotprod16/2, dotprod17/2, dotprod18/2, dotprod19/2, dotprod20/2, dotprod21/2, dotprod22/2, dotprod23/2, dotprod24/2, dotprod25/2, dotprod26/2, dotprod27/2, dotprod28/2, dotprod29/2, dotprod30/2, dotprod31/2, dotprod32/2, dotprod33/2, dotprod34/2, dotprod35/2, dotprod36/2, dotprod37/2, dotprod38/2, dotprod39/2, dotprod40/2, dotprod41/2, dotprod42/2, dotprod43/2, dotprod44/2, dotprod45/2, dotprod46/2, dotprod47/2, dotprod48/2, dotprod49/2, dotprod50/2
  dotprod1/1 -> Mux/1
  "IW{1,1}(2,:)'"/1 -> dotprod2/1
  dotprod2/1 -> Mux/2
  "IW{1,1}(3,:)'"/1 -> dotprod3/1
  dotprod3/1 -> Mux/3
  "IW{1,1}(4,:)'"/1 -> dotprod4/1
  dotprod4/1 -> Mux/4
  "IW{1,1}(5,:)'"/1 -> dotprod5/1
  dotprod5/1 -> Mux/5
  "IW{1,1}(6,:)'"/1 -> dotprod6/1
  dotprod6/1 -> Mux/6
  "IW{1,1}(7,:)'"/1 -> dotprod7/1
  dotprod7/1 -> Mux/7
  "IW{1,1}(8,:)'"/1 -> dotprod8/1
  dotprod8/1 -> Mux/8
  "IW{1,1}(9,:)'"/1 -> dotprod9/1
  dotprod9/1 -> Mux/9
  "IW{1,1}(10,:)'"/1 -> dotprod10/1
  dotprod10/1 -> Mux/10
  "IW{1,1}(11,:)'"/1 -> dotprod11/1
  dotprod11/1 -> Mux/11
  "IW{1,1}(12,:)'"/1 -> dotprod12/1
  dotprod12/1 -> Mux/12
  "IW{1,1}(13,:)'"/1 -> dotprod13/1
  dotprod13/1 -> Mux/13
  "IW{1,1}(14,:)'"/1 -> dotprod14/1
  dotprod14/1 -> Mux/14
  "IW{1,1}(15,:)'"/1 -> dotprod15/1
  dotprod15/1 -> Mux/15
  "IW{1,1}(16,:)'"/1 -> dotprod16/1
  dotprod16/1 -> Mux/16
  "IW{1,1}(17,:)'"/1 -> dotprod17/1
  dotprod17/1 -> Mux/17
  "IW{1,1}(18,:)'"/1 -> dotprod18/1
  dotprod18/1 -> Mux/18
  "IW{1,1}(19,:)'"/1 -> dotprod19/1
  dotprod19/1 -> Mux/19
  "IW{1,1}(20,:)'"/1 -> dotprod20/1
  dotprod20/1 -> Mux/20
  "IW{1,1}(21,:)'"/1 -> dotprod21/1
  dotprod21/1 -> Mux/21
  "IW{1,1}(22,:)'"/1 -> dotprod22/1
  dotprod22/1 -> Mux/22
  "IW{1,1}(23,:)'"/1 -> dotprod23/1
  dotprod23/1 -> Mux/23
  "IW{1,1}(24,:)'"/1 -> dotprod24/1
  dotprod24/1 -> Mux/24
  "IW{1,1}(25,:)'"/1 -> dotprod25/1
  dotprod25/1 -> Mux/25
  "IW{1,1}(26,:)'"/1 -> dotprod26/1
  dotprod26/1 -> Mux/26
  "IW{1,1}(27,:)'"/1 -> dotprod27/1
  dotprod27/1 -> Mux/27
  "IW{1,1}(28,:)'"/1 -> dotprod28/1
  dotprod28/1 -> Mux/28
  "IW{1,1}(29,:)'"/1 -> dotprod29/1
  dotprod29/1 -> Mux/29
  "IW{1,1}(30,:)'"/1 -> dotprod30/1
  dotprod30/1 -> Mux/30
  "IW{1,1}(31,:)'"/1 -> dotprod31/1
  dotprod31/1 -> Mux/31
  "IW{1,1}(32,:)'"/1 -> dotprod32/1
  dotprod32/1 -> Mux/32
  "IW{1,1}(33,:)'"/1 -> dotprod33/1
  dotprod33/1 -> Mux/33
  "IW{1,1}(34,:)'"/1 -> dotprod34/1
  dotprod34/1 -> Mux/34
  "IW{1,1}(35,:)'"/1 -> dotprod35/1
  dotprod35/1 -> Mux/35
  "IW{1,1}(36,:)'"/1 -> dotprod36/1
  dotprod36/1 -> Mux/36
  "IW{1,1}(37,:)'"/1 -> dotprod37/1
  dotprod37/1 -> Mux/37
  "IW{1,1}(38,:)'"/1 -> dotprod38/1
  dotprod38/1 -> Mux/38
  "IW{1,1}(39,:)'"/1 -> dotprod39/1
  dotprod39/1 -> Mux/39
  "IW{1,1}(40,:)'"/1 -> dotprod40/1
  dotprod40/1 -> Mux/40
  "IW{1,1}(41,:)'"/1 -> dotprod41/1
  dotprod41/1 -> Mux/41
  "IW{1,1}(42,:)'"/1 -> dotprod42/1
  dotprod42/1 -> Mux/42
  "IW{1,1}(43,:)'"/1 -> dotprod43/1
  dotprod43/1 -> Mux/43
  "IW{1,1}(44,:)'"/1 -> dotprod44/1
  dotprod44/1 -> Mux/44
  "IW{1,1}(45,:)'"/1 -> dotprod45/1
  dotprod45/1 -> Mux/45
  "IW{1,1}(46,:)'"/1 -> dotprod46/1
  dotprod46/1 -> Mux/46
  "IW{1,1}(47,:)'"/1 -> dotprod47/1
  dotprod47/1 -> Mux/47
  "IW{1,1}(48,:)'"/1 -> dotprod48/1
  dotprod48/1 -> Mux/48
  "IW{1,1}(49,:)'"/1 -> dotprod49/1
  dotprod49/1 -> Mux/49
  "IW{1,1}(50,:)'"/1 -> dotprod50/1
  dotprod50/1 -> Mux/50
  Mux/1 -> "iz{1,1}"/1

== system BLDCMODELTOTALNEURON/Function Fitting Neural Network/Layer 2/Delays 1 ==
  "p{2}" : Inport  PortDimensions=50
      mask Display: e = 0.06;c1 = [120 230 180]/255;c2 = ([120 230 180]+0)/(256+128);c3 = ([120 230 180]+128)/(256+128);patch([0 1 1 0],[0 0 1 1],c1);patch([0 1 1 1-e 1-e 0+e],[0 0 1 1-e 0+e 0+e],c2);patch([0 0 1 1-e 0+e 0+e],[0 1 1 1-e 1-e 0+e],c3);plot([0 1 1 0 0],[0 0 1 1 0]);
  mux : Mux  Inputs=1
      mask Display: e = 0.06;c1 = [120 150 230]/255;c2 = ([120 150 230]+0)/383;c3 = ([120 150 230]+128)/383;patch([0 1 1 0],[0 0 1 1],c1);patch([0 1 1 1-e 1-e 0+e],[0 0 1 1-e 0+e 0+e],c2);patch([0 0 1 1-e 0+e 0+e],[0 1 1 1-e 1-e 0+e],c3);plot([0 1 1 0 0],[0 0 1 1 0]);disp('Mux')
  "pd{2,1}" : Outport
      mask Display: e = 0.06;c1 = [120 230 180]/255;c2 = ([120 230 180]+0)/(256+128);c3 = ([120 230 180]+128)/(256+128);patch([0 1 1 0],[0 0 1 1],c1);patch([0 1 1 1-e 1-e 0+e],[0 0 1 1-e 0+e 0+e],c2);patch([0 0 1 1-e 0+e 0+e],[0 1 1 1-e 1-e 0+e],c3);plot([0 1 1 0 0],[0 0 1 1 0]);
  wires:
  "p{2}"/1 -> mux/1
  mux/1 -> "pd{2,1}"/1
